simulink subsystem "Normal_Forces_and_Moments"  (R2024b)
settings: Solver=VariableStepAuto  StartTime=0.0  StopTime=10.0  RelTol=1e-3
undefined symbols (not defined in the file or in its folder): CNa_body, CNa_canard, CNa_data_aoa, CNa_data_mach, CNa_fins, CNa_input_aoa, CNa_input_mach, CNa_nosecone, CNa_tail, OR_cg, sim_time, x_cp_tot, x_pos_bodytube, x_pos_canard, x_pos_fins, x_pos_nosecone, x_pos_tail
libraries: sharedutil x1
settings Model: Creator=joedo  LastModifiedBy=finnb

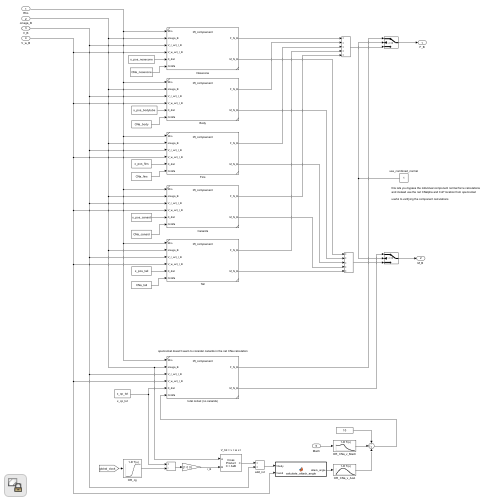
[thumbnail: Simulink's stored preview of the top-level diagram]
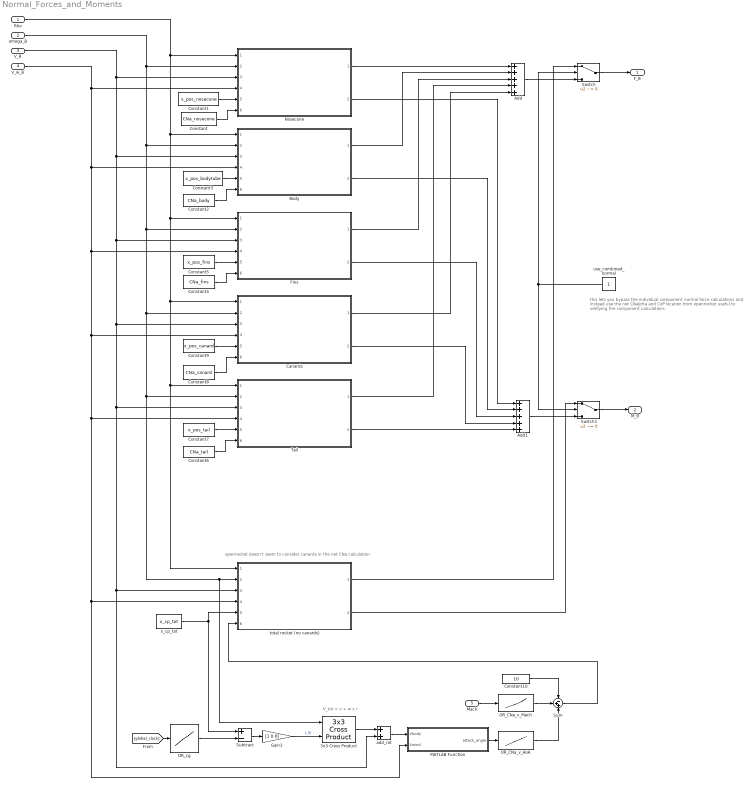
== system Normal_Forces_and_Moments ==
  note: openrocket doesn't seem to consider canards in the net CNa calculation
  note: this lets you bypass the individual component normal force calculations
      | and instead use the net CNalpha and CoP location from openrocket
      |
      | useful to verifying the component calculations
  note: V_tot = v + w x r
  Rho : Inport
  omega_B : Inport  Port=2
  "V_B " : Inport  Port=3
  V_w_B : Inport  Port=4
  Mach : Inport  Port=5
  3x3 Cross Product : sharedutil/3x3 Cross Product  aMode=aMode
  Add : Sum  Inputs=+++++
  Add1 : Sum  Inputs=+++++
  Body : Subsystem  ReferencedSubsystem=lift_compoenent
  Canards : Subsystem  ReferencedSubsystem=lift_compoenent
  Constant : Constant  Value=CNa_nosecone
  Constant1 : Constant  Value=x_pos_nosecone
  Constant10 : Constant  Value=10
  Constant2 : Constant  Value=CNa_body
  Constant3 : Constant  Value=x_pos_bodytube
  Constant4 : Constant  Value=CNa_fins
  Constant5 : Constant  Value=x_pos_fins
  Constant6 : Constant  Value=CNa_tail
  Constant7 : Constant  Value=x_pos_tail
  Constant8 : Constant  Value=CNa_canard
  Constant9 : Constant  Value=x_pos_canard
  Fins : Subsystem  ReferencedSubsystem=lift_compoenent
  Gain3 : Gain  Gain=[1 0 0]
  MATLAB Function : MATLAB Function  TreatAsAtomicUnit=on
  Nosecone : Subsystem  ReferencedSubsystem=lift_compoenent
  OR_CNa_v_AoA : Lookup_n-D  NumberOfTableDimensions=1  BreakpointsForDimension1=CNa_input_aoa  Table=CNa_data_aoa  InternalRulePriority=Speed  RndMeth=Simplest
  OR_CNa_v_Mach : Lookup_n-D  NumberOfTableDimensions=1  BreakpointsForDimension1=CNa_input_mach  Table=CNa_data_mach  InternalRulePriority=Speed  RndMeth=Simplest
  OR_cg : Lookup_n-D  NumberOfTableDimensions=1  BreakpointsForDimension1=sim_time  Table=OR_cg  InternalRulePriority=Speed  RndMeth=Simplest
  Subtract : Sum  Inputs=+-
  Sum : Sum  Inputs=-++
  Switch : Switch  Criteria=u2 ~= 0  SaturateOnIntegerOverflow=off  InputSameDT=off
  Switch1 : Switch  Criteria=u2 ~= 0  SaturateOnIntegerOverflow=off  InputSameDT=off
  Tail : Subsystem  ReferencedSubsystem=lift_compoenent
  add_rot : Sum
  total rocket (no canards) : Subsystem  ReferencedSubsystem=lift_compoenent
  use_combined_normal : Constant
  x_cp_tot : Constant  Value=x_cp_tot
  "F_B " : Outport  VectorParamsAs1DForOutWhenUnconnected=off
  "M_B " : Outport  Port=2  VectorParamsAs1DForOutWhenUnconnected=off
  wires:
  V_w_B/1 -> total rocket (no canards)/4, MATLAB Function/2(Vwind), Tail/4, Canards/4, Fins/4, Body/4, Nosecone/4
  Constant8/1 -> Canards/6
  Constant9/1 -> Canards/5
  Constant6/1 -> Tail/6
  Constant7/1 -> Tail/5
  Constant4/1 -> Fins/6
  Constant5/1 -> Fins/5
  Constant3/1 -> Body/5
  Constant2/1 -> Body/6
  Nosecone/2 -> Add1/1
  Nosecone/1 -> Add/1
  Constant1/1 -> Nosecone/5
  Constant/1 -> Nosecone/6
  Canards/2 -> Add1/4
  Canards/1 -> Add/5
  Tail/2 -> Add1/5
  Tail/1 -> Add/4
  Fins/2 -> Add1/3
  Fins/1 -> Add/3
  Body/2 -> Add1/2
  Body/1 -> Add/2
  Add/1 -> Switch/3
  Add1/1 -> Switch1/3
  Rho/1 -> Nosecone/1, Body/1, total rocket (no canards)/1, Tail/1, Canards/1, Fins/1
  "V_B "/1 -> Nosecone/3, add_rot/2, total rocket (no canards)/3, Tail/3, Canards/3, Fins/3, Body/3
  use_combined_normal/1 -> Switch/2, Switch1/2
  Switch/1 -> "F_B "/1
  total rocket (no canards)/1 -> Switch/1
  Switch1/1 -> "M_B "/1
  total rocket (no canards)/2 -> Switch1/1
  Mach/1 -> OR_CNa_v_Mach/1
  OR_CNa_v_Mach/1 -> Sum/2
  OR_CNa_v_AoA/1 -> Sum/3
  MATLAB Function/1(attack_angle) -> OR_CNa_v_AoA/1
  Gain3/1 -> 3x3 Cross Product/2  "r_B"
  omega_B/1 -> 3x3 Cross Product/1, total rocket (no canards)/2, Tail/2, Canards/2, Fins/2, Body/2, Nosecone/2
  OR_cg/1 -> Subtract/2
  [global_clock] -> OR_cg/1
  Subtract/1 -> Gain3/1
  x_cp_tot/1 -> Subtract/1, total rocket (no canards)/5
  3x3 Cross Product/1 -> add_rot/1
  add_rot/1 -> MATLAB Function/1(Vbody)
  Sum/1 -> total rocket (no canards)/6
  Constant10/1 -> Sum/1

== matlab function Normal_Forces_and_Moments/MATLAB Function ==
  data: Vbody input; attack_angle output; Vwind input
function attack_angle  = calculate_attack_angle(Vbody, Vwind)
%% Wind Calcs
% Body relative velocity
Vrel = Vbody - Vwind;
% Body relative velocity magnitude
Vrel_mag = norm(Vrel);
VrelMagYZ = (Vrel(3) ^ 2 + Vrel(2) ^ 2)^0.5;

if Vrel_mag ~= 0 % prevent division by 0
    attack_angle = asin(VrelMagYZ/Vrel_mag);
else
    attack_angle = 0;
end
